simulink model "model1"  (R2022a)
settings: Solver=VariableStepAuto  StartTime=0.0  StopTime=10.0  RelTol=1e-3
settings Model: Creator=tano-  LastModifiedBy=tano-

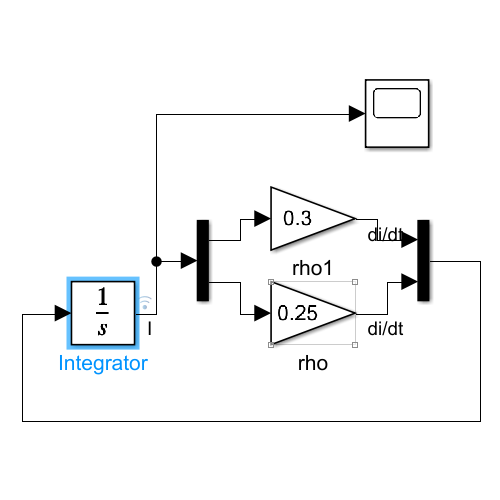
[thumbnail: Simulink's stored preview of the top-level diagram]
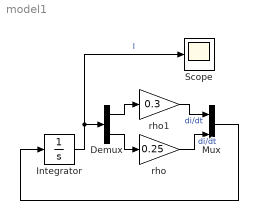
== system model1 ==
  Demux : Demux  Outputs=2
  Integrator : Integrator  InitialCondition=[1 1]
  Mux : Mux  Inputs=2
  Scope : Scope
  rho : Gain  Gain=0.25
  rho1 : Gain  Gain=0.3
  wires:
  Integrator/1 -> Scope/1, Demux/1  "I"
  Demux/1 -> rho1/1
  Demux/2 -> rho/1
  rho1/1 -> Mux/1  "di/dt"
  rho/1 -> Mux/2  "di/dt"
  Mux/1 -> Integrator/1
